simulink model "chap04_02_18_mdl"  (R2013b)
settings: Solver=ode45  StartTime=0.0  StopTime=10.0  RelTol=1e-3
libraries: simulink_extras x1
settings Model: Creator=Administrator  LastModifiedBy=sunzx.fnst

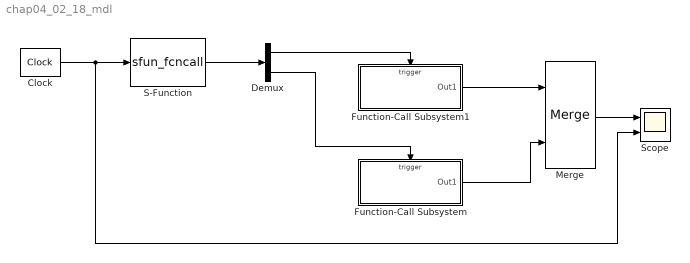
== system chap04_02_18_mdl ==
  Clock : simulink_extras/Flip Flops/Clock  period=2
  Demux : Demux  Outputs=2
  Function-Call Subsystem : Subsystem  TreatAsAtomicUnit=on
  Function-Call Subsystem1 : Subsystem  TreatAsAtomicUnit=on
  Merge : Merge
  S-Function : S-Function  FunctionName=sfun_fcncall  EnableBusSupport=off
  Scope : Scope  NumInputPorts=2
      settings: YMin=-5~-5  YMax=5~5
  wires:
  Clock/1 -> Scope/2, S-Function/1
  S-Function/1 -> Demux/1
  Demux/2 -> Function-Call Subsystem/Trigger
  Demux/1 -> Function-Call Subsystem1/Trigger
  Function-Call Subsystem1/1(Out1) -> Merge/1
  Function-Call Subsystem/1(Out1) -> Merge/2
  Merge/1 -> Scope/1

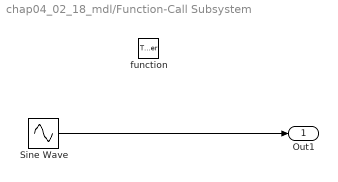
== system chap04_02_18_mdl/Function-Call Subsystem ==
  function : TriggerPort  TriggerType=function-call
  Sine Wave : Sin
  Out1 : Outport
  wires:
  Sine Wave/1 -> Out1/1

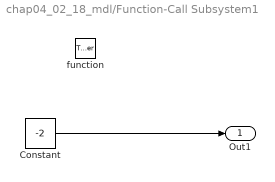
== system chap04_02_18_mdl/Function-Call Subsystem1 ==
  function : TriggerPort  TriggerType=function-call
  Constant : Constant  Value=-2
  Out1 : Outport
  wires:
  Constant/1 -> Out1/1
